simulink model "controlled_V_three_phase_full_model"  (Simulink 7.7)
settings: Solver=ode45  StartTime=0.0  StopTime=10.0  RelTol=1e-3
libraries: powerlib x3
settings Model: Creator=s0237326  LastModifiedBy=s0237326
settings OptimizationCC: InlineParams=on  EnhancedBackFolding=on

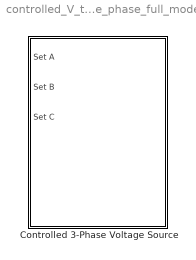
== system controlled_V_three_phase_full_model ==
  Controlled 3-Phase Voltage Source : Subsystem

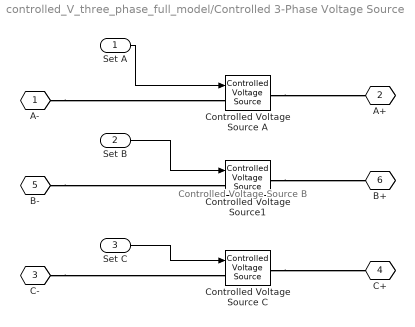
== system controlled_V_three_phase_full_model/Controlled 3-Phase Voltage Source ==
  note: Controlled Voltage Source B
  Set A : Inport  PortDimensions=1
  Set B : Inport  Port=2  PortDimensions=1
  Set C : Inport  Port=3  PortDimensions=1
  Controlled Voltage Source A : powerlib/Electrical Sources/Controlled Voltage Source  SystemSampleTime=-1  Initialize=on  Source_Type=AC  Amplitude=0  Phase=0  Frequency=0  Measurements=None
  Controlled Voltage Source C : powerlib/Electrical Sources/Controlled Voltage Source  SystemSampleTime=-1  Initialize=on  Source_Type=AC  Amplitude=0  Phase=0  Frequency=0  Measurements=None
  Controlled Voltage Source1 : powerlib/Electrical Sources/Controlled Voltage Source  SystemSampleTime=-1  Initialize=on  Source_Type=AC  Amplitude=0  Phase=0  Frequency=0  Measurements=None
  A- : PMIOPort  Tag=PMCPort  Port=1  Side=Left
  A+ : PMIOPort  Tag=PMCPort  Port=2  Side=Right
  C- : PMIOPort  Tag=PMCPort  Port=3  Side=Left
  C+ : PMIOPort  Tag=PMCPort  Port=4  Side=Right
  B- : PMIOPort  Tag=PMCPort  Port=5  Side=Left
  B+ : PMIOPort  Tag=PMCPort  Port=6  Side=Right
  wires:
  Set C/1 -> Controlled Voltage Source C/1
  Set B/1 -> Controlled Voltage Source1/1
  Set A/1 -> Controlled Voltage Source A/1
  connections:
  A-/RConn1 -- Controlled Voltage Source A/LConn1
  Controlled Voltage Source A/RConn1 -- A+/RConn1
  C-/RConn1 -- Controlled Voltage Source C/LConn1
  Controlled Voltage Source C/RConn1 -- C+/RConn1
  B-/RConn1 -- Controlled Voltage Source1/LConn1
  Controlled Voltage Source1/RConn1 -- B+/RConn1
